simulink model "Boat_NonLinear_Actuator"  (R2020a)
settings: Solver=ode23  StartTime=0.0  StopTime=20  MaxStep=0.001  RelTol=1e-3
libraries: simulink x2
settings Model: NumberOfSteps=10  Creator=micro microndas  LastModifiedBy=micro microndas

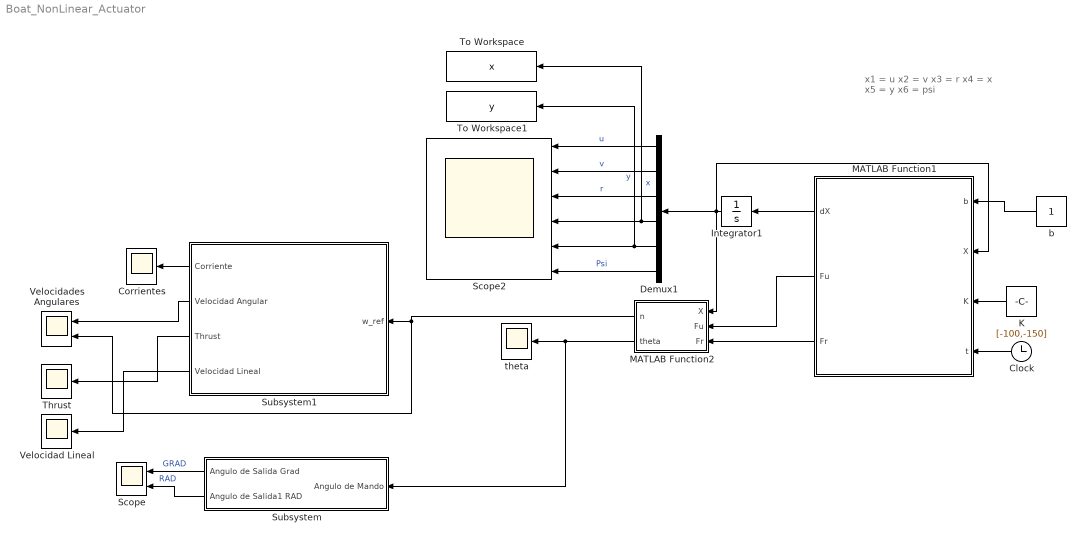
== system Boat_NonLinear_Actuator ==
  note: x1 = u
      | x2 = v
      | x3 = r
      | x4 = x
      | x5 = y
      | x6 = psi
  Clock : Clock
  "Corrientes " : Scope
  Demux1 : Demux  Outputs=6
  Integrator1 : Integrator  InitialCondition=[0 0 0 0 0 -pi/4]
  K : Constant  Value=[-100,-150]
  MATLAB Function1 : MATLAB Function  TreatAsAtomicUnit=on
  MATLAB Function2 : MATLAB Function  TreatAsAtomicUnit=on
  Scope : Scope  NumInputPorts=2
  Scope2 : Scope  NumInputPorts=6
  Subsystem : Subsystem
  Subsystem1 : Subsystem
  Thrust : Scope
  To Workspace : ToWorkspace  VariableName=x  SampleTime=-1
      settings: Save2DSignal=2-D array (concatenate along first dimension)
  To Workspace1 : ToWorkspace  VariableName=y  SampleTime=-1
      settings: Save2DSignal=2-D array (concatenate along first dimension)
  Velocidad Lineal : Scope
  "Velocidades Angulares " : Scope  NumInputPorts=2
  b : Constant
  theta : Scope
  wires:
  MATLAB Function1/1(dX) -> Integrator1/1
  b/1 -> MATLAB Function1/1(b)
  K/1 -> MATLAB Function1/3(K)
  Integrator1/1 -> MATLAB Function1/2(X), MATLAB Function2/1(X), Demux1/1
  Demux1/1 -> Scope2/1  "u"
  Demux1/2 -> Scope2/2  "v"
  Demux1/3 -> Scope2/3  "r"
  Demux1/4 -> Scope2/4, To Workspace/1  "x"
  Demux1/5 -> Scope2/5, To Workspace1/1  "y"
  Demux1/6 -> Scope2/6  "Psi"
  MATLAB Function1/3(Fr) -> MATLAB Function2/3(Fr)
  MATLAB Function1/2(Fu) -> MATLAB Function2/2(Fu)
  Subsystem1/2(Velocidad Angular) -> "Velocidades Angulares "/1
  Subsystem1/3(Thrust) -> Thrust/1
  Subsystem1/1(Corriente) -> "Corrientes "/1
  MATLAB Function2/1(n) -> "Velocidades Angulares "/2, Subsystem1/1(w_ref)
  MATLAB Function2/2(theta) -> Subsystem/1(Angulo de Mando), theta/1
  Clock/1 -> MATLAB Function1/4(t)
  Subsystem/1(Angulo de Salida Grad) -> Scope/1  "GRAD"
  Subsystem/2(Angulo de Salida1 RAD) -> Scope/2  "RAD"
  Subsystem1/4(Velocidad Lineal) -> Velocidad Lineal/1

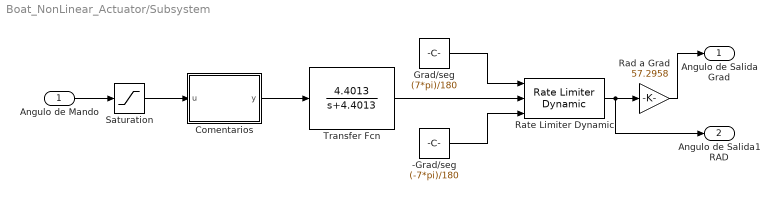
== system Boat_NonLinear_Actuator/Subsystem ==
  Angulo de Mando : Inport
  -Grad/seg : Constant  Value=(-7*pi)/180
  Comentarios : MATLAB Function  TreatAsAtomicUnit=on
  Grad/seg : Constant  Value=(7*pi)/180
  Rad a Grad : Gain  Gain=57.2958
  Rate Limiter Dynamic : simulink/Discontinuities/Rate Limiter Dynamic
  Saturation : Saturate  UpperLimit=pi/2  LowerLimit=-pi/2
  Transfer Fcn : TransferFcn  Numerator=[4.4013]  Denominator=[1 4.4013]
  Angulo de Salida Grad : Outport
  Angulo de Salida1 RAD : Outport  Port=2
  wires:
  Transfer Fcn/1 -> Rate Limiter Dynamic/2
  Grad/seg/1 -> Rate Limiter Dynamic/1
  -Grad/seg/1 -> Rate Limiter Dynamic/3
  Rate Limiter Dynamic/1 -> Angulo de Salida1 RAD/1, Rad a Grad/1
  Rad a Grad/1 -> Angulo de Salida Grad/1
  Comentarios/1(y) -> Transfer Fcn/1
  Saturation/1 -> Comentarios/1(u)
  Angulo de Mando/1 -> Saturation/1

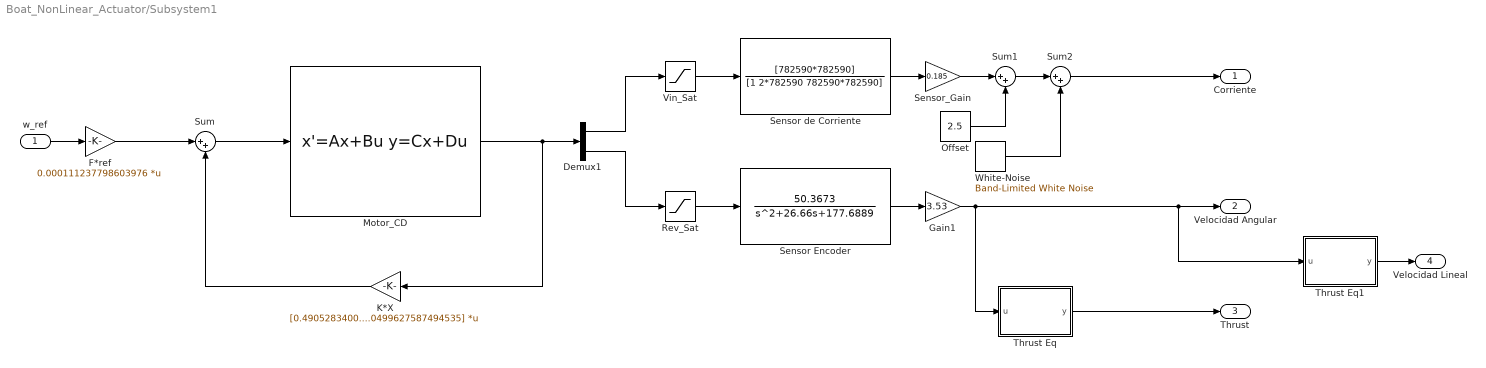
== system Boat_NonLinear_Actuator/Subsystem1 ==
  w_ref : Inport
  Demux1 : Demux  Outputs=2
  F*ref : Gain  Gain=0.000111237798603976  Multiplication=Matrix(K*u)
  Gain1 : Gain  Gain=3.53
  K*X : Gain  Gain=[0.490528340000000, 0.0499627587494535]  Multiplication=Matrix(K*u)
  Motor_CD : StateSpace  A=[-333.333333333333, -33.3333333333333;215.754000000000, -1.68556000000000]  B=[666.666666666667; 0]  C=eye(2)  D=[0;0]  InitialCondition=0  ContinuousStateAttributes={'i_t', 'w_t'}
  Offset : Constant  Value=2.5
  Rev_Sat : Saturate  UpperLimit=7500  LowerLimit=0
  Sensor Encoder : TransferFcn  Numerator=[50.3673]  Denominator=[1 26.66 177.6889]  ContinuousStateAttributes='Position'
  "Sensor de Corriente " : TransferFcn  Numerator=[782590*782590]  Denominator=[1 2*782590 782590*782590]  ContinuousStateAttributes='Corriente'
  Sensor_Gain : Gain  Gain=0.185
  Sum : Sum  Inputs=|++
  Sum1 : Sum  Inputs=|++
  Sum2 : Sum  Inputs=|++
  Thrust Eq : MATLAB Function  TreatAsAtomicUnit=on
  Thrust Eq1 : MATLAB Function  TreatAsAtomicUnit=on
  Vin_Sat : Saturate  UpperLimit=5  LowerLimit=-5
  White-Noise : simulink/Sources/Band-Limited White Noise  Cov=[1e-8]  Ts=0.001  seed=[23341]
  Corriente : Outport
  Velocidad Angular : Outport  Port=2
  Thrust : Outport  Port=3
  Velocidad Lineal : Outport  Port=4
  wires:
  Rev_Sat/1 -> Sensor Encoder/1
  "Sensor de Corriente "/1 -> Sensor_Gain/1
  Demux1/2 -> Rev_Sat/1
  Gain1/1 -> Thrust Eq1/1(u), Velocidad Angular/1, Thrust Eq/1(u)
  Sum1/1 -> Sum2/1
  K*X/1 -> Sum/2
  Demux1/1 -> Vin_Sat/1
  Motor_CD/1 -> K*X/1, Demux1/1
  White-Noise/1 -> Sum2/2
  Thrust Eq/1(y) -> Thrust/1
  Sum/1 -> Motor_CD/1
  Offset/1 -> Sum1/2
  F*ref/1 -> Sum/1
  Sum2/1 -> Corriente/1
  Sensor_Gain/1 -> Sum1/1
  Sensor Encoder/1 -> Gain1/1
  Vin_Sat/1 -> "Sensor de Corriente "/1
  w_ref/1 -> F*ref/1
  Thrust Eq1/1(y) -> Velocidad Lineal/1

== matlab function Boat_NonLinear_Actuator/MATLAB Function1 ==
  data: b input; X input; dX output; K input; Fu output; Fr output; t input
function [dX,Fu, Fr] = fcn(b, X, K, t)

k1 = K(1);
k2 = K(2);

y1_ref = -12;
y2_ref = 26;

x4_ref = y1_ref;
x5_ref = y2_ref;

dx4_ref = 0;
dx5_ref = 0;

ddx4_ref = 0;
ddx5_ref = 0;

e1 =  [x4_ref;
       x5_ref] - [X(4);
                  X(5)];
d_e1 = [dx4_ref; 
        dx5_ref ] - [ cos(X(6)), -sin(X(6)); 
                      sin(X(6)), cos(X(6))]*[X(1);X(2)];

x_ref = [ cos(X(6)), sin(X(6));
             -sin(X(6)), cos(X(6))]*(  [dx4_ref; 
                                        dx5_ref ]  - k1*e1);

dx_ref = [ -sin(X(6)), cos(X(6));
              -cos(X(6)), -sin(X(6))]*( [dx4_ref; 
                                         dx5_ref ] -e1*k1 ) + [ cos(X(6)), sin(X(6));
                                                               -sin(X(6)), cos(X(6))]*( [ddx4_ref;
                                                                                         ddx5_ref] -d_e1*k1 );
e2 = [x_ref(1);
      x_ref(2)] - [X(1);
                 X(2)];
             
u = inv([0.0185, 0;
            0, 0.0110*b])*( [dx_ref(1);
                             dx_ref(2)] - [-0.2775, 0;
                                         0.7*X(3), 0.2083]*[X(1);
                                                            X(2)] -e2*k2 );
dX = [-0.2775*X(1);0.7*X(1)*X(3) + 0.2083*X(2);0.7*X(1)*X(3) + 0.2083*X(2);X(1)*cos(X(6))-X(2)*sin(X(6));X(1)*sin(X(6)) + X(2)*cos(X(6));X(3)] + [[0.0185, 0;0,0.011*b];0, 0.011*b;0, 0;0, 0;0, 0]*u;

Fu = u(1);
Fr = u(2);

== matlab function Boat_NonLinear_Actuator/Subsystem/Comentarios ==
  data: u input; y output
function y = fcn(u)

%Kg' = Kg*L / U
    %Kg = Maximo giro del timon / error maximo
        %error maximo
        %Maximo giro del timon
    %L = Eslora / Longitud del buque
        %390.00 𝑓𝑡 
        %118.872 mts
    %U = Velocidad del buque
        %15 nudo nautico
        %7.7166 m/s

y = u;

== matlab function Boat_NonLinear_Actuator/MATLAB Function2 ==
  data: X input; Fu input; n output; Fr input; theta output
function [n, theta] = fcn(X, Fu, Fr)

T1 = 0.26;  T2= 0.1; b = 1; 

V = sqrt( X(1)^2 + (X(3)*b)^2 );
F = sqrt( Fu^2 + Fr^2 ); 

theta = atan(-Fr/Fu);
n =( T1*V + sqrt( (T2*V)^2 + 4*F*T2)) / (2*T1^2);

== matlab function Boat_NonLinear_Actuator/Subsystem1/Thrust Eq ==
  data: u input; y output
function y = Thrust_Eq(u)

% Valores para propela
    % Thrust = Thrust_Coef*( density*Rev*Rev*Diam*Diam*Diam*Diam )

    Thrust_Coef = 0.014;
    density = 1e3; %kg/mts*mts*mts
    Diam = 0.2; %mts
    
y = ( Thrust_Coef )*( density )*( u^2 )*( Diam^4 ) ;

== matlab function Boat_NonLinear_Actuator/Subsystem1/Thrust Eq1 ==
  data: u input; y output
function y = Vel_Lineal(u)

r = 0.1; %mts
    
y = u*r;
